simulink model "TestMotores"  (R2024b)
settings: Solver=FixedStepAuto  StartTime=0.0  StopTime=inf  RelTol=1e-3  EnableMultiTasking=on
settings Model: ExtModeTrigDuration=2  Creator=Chenfu  LastModifiedBy=lucia
settings SolverCC: AutoInsertRateTranBlk=on
settings OptimizationCC: DefaultParameterBehavior=Inlined  EnhancedBackFolding=on  PassReuseOutputArgsAs=Individual arguments  ZeroExternalMemoryAtStartup=off  ZeroInternalMemoryAtStartup=off  MaxStackSize=64  OptimizeBlockOrder=speed  DifferentSizesBufferReuse=on  OptimizationCustomize=off  EfficientTunableParamExpr=on
settings DebuggingCC: ParameterTunabilityLossMsg=error
settings HardwareCC: ProdBitPerInt=16  ProdBitPerPointer=16  ProdBitPerSizeT=16  ProdBitPerPtrDiffT=16  ProdLargestAtomicFloat=None  ProdWordSize=8  ProdHWDeviceType=Atmel->AVR
settings SFSimCC: MATLABDynamicMemAlloc=off
settings RTWCC: Description=Embedded Coder  SystemTargetFile=ert.tlc  HardwareBoard=Arduino Mega 2560  TemplateMakefile=ert_default_tmf  Toolchain=Arduino AVR  BuildConfiguration=Faster Runs  GPUComputeCapability=3.5
settings CodeAppCC: ForceParamTrailComments=on  IgnoreCustomStorageClasses=off  OperatorAnnotations=on  SimulinkDataObjDesc=on  SFDataObjDesc=on  InsertBlockDesc=on
settings ERTTargetCC: SupportContinuousTime=on  SupportNonInlinedSFcns=on  SupportVariableSizeSignals=on  ExtModeTransport=3  ExtModeStaticAlloc=on  ExtModeAutomaticAllocSize=off  ExtModeStaticAllocSize=2048  ExtModeMexFile=ext_xcp  ExtModeIntrfLevel=Level2 - Open

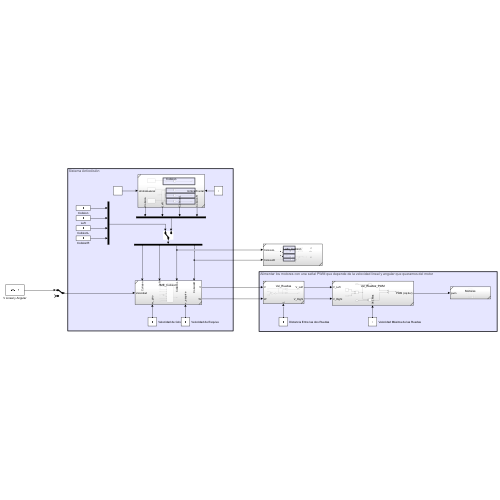
[thumbnail: Simulink's stored preview of the top-level diagram]
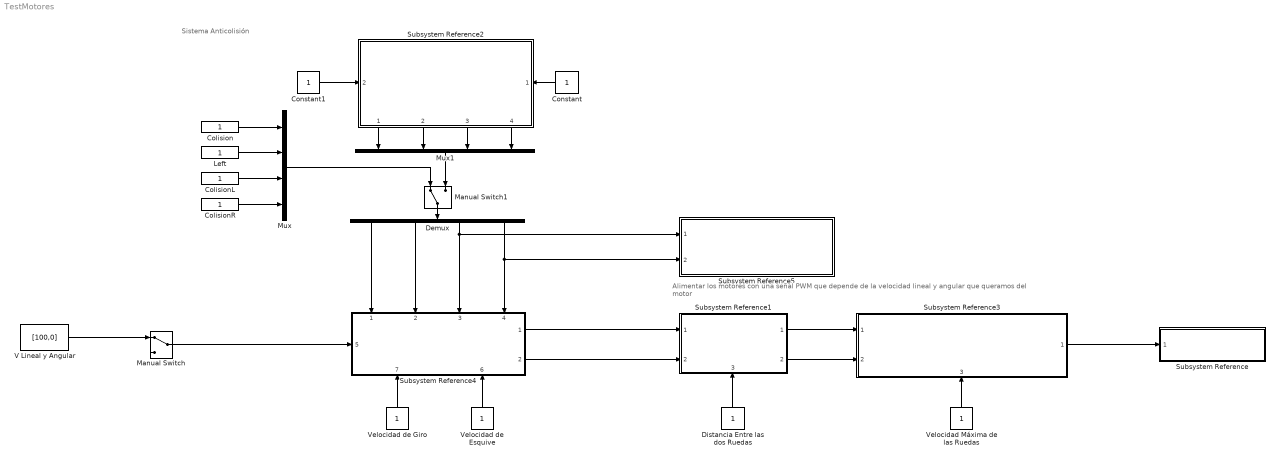
== system TestMotores ==
  note: Sistema Anticolisión
  note: Alimentar los motores con una señal PWM que depende de la velocidad lineal y angular que queramos del motor
  Colision : Constant
  ColisionL : Constant
  ColisionR : Constant
  Constant : Constant
  Constant1 : Constant
  Demux : Demux
  Distancia Entre las dos Ruedas : Constant
  Left : Constant
  Manual Switch : ManualSwitch
  Manual Switch1 : ManualSwitch
  Mux : Mux
  Mux1 : Mux
  Subsystem Reference : Subsystem  ReferencedSubsystem=Motores
  Subsystem Reference1 : Subsystem  ReferencedSubsystem=Vel_Ruedas
      settings: PortSchema="{\"entries\":[{\"content\":{\"sides\":[{\"content\":{\"connectorIds\":[\"In1\",\"In2\"]},\"type\":\"ConnectorPlacement.EquallySpacedRectSide\",\"uuid\":\"d84dcb5e-3d1f-491a-afee-794ad5554a2e\"},{\"content\":{\"connectorIds\":[\"Out1\",\"Out2\"],\"side\":\"RIGHT\"},\"type\":\"ConnectorPlacement.EquallySpacedRectSide\",\"uuid\":\"a0418b62-0e7f-41b6-9229-39e60bbbb316\"},{\"content\":{\"side\":\"TOP\"},\"type\":\"ConnectorPlacement.EquallySpacedRectSide\",\"uuid\":\"a2fa68ab-86c2-485e-93ce-d55ad9856492\"},{\"content\":{\"connectorIds\":[\"In3\"],\"side\":\"BOTTOM\"},\"type\":\"ConnectorPlacement.EquallySpacedRectSide\",\"uuid\":\"b1e52622-770d-4fba-ba7c-301b5de809e8\"}]},\"type\":\"ConnectorPlacement.EquallySpacedConnector\",\"uuid\":\"dfc2f15c-5eb1-4bff-a24d-1444b10fabc2\"}],\"packageUris\":[\"http://schema.mathworks.com/mf0/Connector/R2020b\"],\"version\":\"1.0\"}"
  Subsystem Reference2 : Subsystem  ReferencedSubsystem=Colision
      settings: PortSchema="{\"entries\":[{\"content\":{\"sides\":[{\"content\":{\"connectorIds\":[\"In2\"]},\"type\":\"ConnectorPlacement.EquallySpacedRectSide\",\"uuid\":\"408cd73f-1857-4da1-ae96-c05435cac705\"},{\"content\":{\"connectorIds\":[\"In1\"],\"side\":\"RIGHT\"},\"type\":\"ConnectorPlacement.EquallySpacedRectSide\",\"uuid\":\"c558c647-ecf2-46f4-93b3-68ffd7ab6733\"},{\"content\":{\"side\":\"TOP\"},\"type\":\"ConnectorPlacement.EquallySpacedRectSide\",\"uuid\":\"d0f1560b-589e-4add-97c7-7e558b50eec2\"},{\"content\":{\"connectorIds\":[\"Out1\",\"Out2\",\"Out3\",\"Out4\"],\"side\":\"BOTTOM\"},\"type\":\"ConnectorPlacement.EquallySpacedRectSide\",\"uuid\":\"e27d42a1-23f8-4a2a-9b17-20a6cb6458d1\"}]},\"type\":\"ConnectorPlacement.EquallySpacedConnector\",\"uuid\":\"6a4a7c7e-833b-4492-9d12-ab73c24b9d4d\"}],\"packageUris\":[\"http://schema.mathworks.com/mf0/Connector/R2020b\"],\"version\":\"1.0\"}"
  Subsystem Reference3 : Subsystem  ReferencedSubsystem=Vel_Ruedas_PWM
      settings: PortSchema="{\"entries\":[{\"content\":{\"sides\":[{\"content\":{\"connectorIds\":[\"In1\",\"In2\"]},\"type\":\"ConnectorPlacement.EquallySpacedRectSide\",\"uuid\":\"d4b2428c-e0ec-438f-b8c2-c34143e0f9eb\"},{\"content\":{\"connectorIds\":[\"Out1\"],\"side\":\"RIGHT\"},\"type\":\"ConnectorPlacement.EquallySpacedRectSide\",\"uuid\":\"3bf3e00d-c923-4f77-a6ba-e5133a80a898\"},{\"content\":{\"side\":\"TOP\"},\"type\":\"ConnectorPlacement.EquallySpacedRectSide\",\"uuid\":\"e66e75c4-3d83-4196-961e-523874c887b8\"},{\"content\":{\"connectorIds\":[\"In3\"],\"side\":\"BOTTOM\"},\"type\":\"ConnectorPlacement.EquallySpacedRectSide\",\"uuid\":\"87f1b5fc-600e-4f11-b10b-7f5345f30bd5\"}]},\"type\":\"ConnectorPlacement.EquallySpacedConnector\",\"uuid\":\"27e1c138-7895-410b-a3ac-a83d4beefda8\"}],\"packageUris\":[\"http://schema.mathworks.com/mf0/Connector/R2020b\"],\"version\":\"1.0\"}"
  Subsystem Reference4 : Subsystem  ReferencedSubsystem=ME_Colision
      settings: PortSchema="{\"entries\":[{\"content\":{\"sides\":[{\"content\":{\"connectorIds\":[\"In5\"]},\"type\":\"ConnectorPlacement.EquallySpacedRectSide\",\"uuid\":\"fd240e3c-6394-4405-8519-0479f77d2d36\"},{\"content\":{\"connectorIds\":[\"Out1\",\"Out2\"],\"side\":\"RIGHT\"},\"type\":\"ConnectorPlacement.EquallySpacedRectSide\",\"uuid\":\"6add68b4-b4ce-48ef-b5c5-69d1ef184884\"},{\"content\":{\"connectorIds\":[\"In1\",\"In2\",\"In3\",\"In4\"],\"side\":\"TOP\"},\"type\":\"ConnectorPlacement.EquallySpacedRectSide\",\"uuid\":\"65e91425-4ef2-48e9-b7a9-d3b65ea8e822\"},{\"content\":{\"connectorIds\":[\"In7\",\"In6\"],\"side\":\"BOTTOM\"},\"type\":\"ConnectorPlacement.EquallySpacedRectSide\",\"uuid\":\"6a9c56c5-dfed-4d72-bc8b-a85f8cbcc4c7\"}]},\"type\":\"ConnectorPlacement.EquallySpacedConnector\",\"uuid\":\"4936f7de-35b8-4d13-b291-96fbfb671eec\"}],\"packageUris\":[\"http://schema.mathworks.com/mf0/Connector/R2020b\"],\"version\":\"1.0\"}"
  Subsystem Reference5 : Subsystem  ReferencedSubsystem=Leds_Colision
  V Lineal y Angular : Constant  Value=[100,0]
  Velocidad Máxima de las Ruedas : Constant
  Velocidad de Esquive : Constant
  Velocidad de Giro : Constant
  wires:
  Subsystem Reference3/1 -> Subsystem Reference/1
  Subsystem Reference1/1 -> Subsystem Reference3/1
  Subsystem Reference1/2 -> Subsystem Reference3/2
  Velocidad Máxima de las Ruedas/1 -> Subsystem Reference3/3
  Distancia Entre las dos Ruedas/1 -> Subsystem Reference1/3
  Subsystem Reference4/1 -> Subsystem Reference1/1
  Subsystem Reference4/2 -> Subsystem Reference1/2
  Constant/1 -> Subsystem Reference2/1
  Constant1/1 -> Subsystem Reference2/2
  Manual Switch/1 -> Subsystem Reference4/5
  V Lineal y Angular/1 -> Manual Switch/1
  Subsystem Reference2/1 -> Mux1/1
  Subsystem Reference2/2 -> Mux1/2
  Mux1/1 -> Manual Switch1/2
  Manual Switch1/1 -> Demux/1
  ColisionR/1 -> Mux/4
  ColisionL/1 -> Mux/3
  Colision/1 -> Mux/1
  Left/1 -> Mux/2
  Mux/1 -> Manual Switch1/1
  Velocidad de Esquive/1 -> Subsystem Reference4/6
  Velocidad de Giro/1 -> Subsystem Reference4/7
  Demux/1 -> Subsystem Reference4/1
  Demux/2 -> Subsystem Reference4/2
  Demux/3 -> Subsystem Reference4/3, Subsystem Reference5/1
  Demux/4 -> Subsystem Reference4/4, Subsystem Reference5/2
  Subsystem Reference2/3 -> Mux1/3
  Subsystem Reference2/4 -> Mux1/4
